simulink model "single_tank"  (R2023b)
settings: Solver=ode45  StartTime=0.0  StopTime=199.9  RelTol=1e-3  EnableMultiTasking=on
values from neighbouring files (symbols this model uses):
  A1 = 0.0154    [INIT.m]
  Cvo = 1.59640*1e-4    (= 0.00015964)    [INIT.m]
  h1c = 0.5    [INIT.m]
  h1c_0 = 0    [INIT.m]
  h1max = 0.6    [INIT.m]
  Ki = 5*1e-6    (= 5e-06)    [INIT.m]
  Kp = 1e-3    (= 0.001)    [INIT.m]
  Qf1 = 1e-4    (= 0.0001)    [INIT.m]    (also in extract_data.m = 5e-5*randn + 1e-4)
  Qf2 = 1e-4    (= 0.0001)    [INIT.m]    (also in extract_data.m = 5e-5*randn + 1e-4)
  Qpmax = 1e-2    (= 0.01)    [INIT.m]
  rate_noise_mQp = 1e-6    (= 1e-06)    [INIT.m]
  rate_noise_mUp = 1e-6    (= 1e-06)    [INIT.m]
  rate_noise_my1 = 1e-6    (= 1e-06)    [INIT.m]
  Te = 1    [INIT.m]
  yo = 0    [INIT.m]
settings Model: Creator=upcnet  LastModifiedBy=Plambeck
settings SolverCC: AlgebraicLoopSolver=TrustRegion
settings DataIOCC: LimitDataPoints=on  SaveFormat=Array  SignalLoggingSaveFormat=ModelDataLogs  ReturnWorkspaceOutputs=off  SignalLoggingName=sigsOut
settings OptimizationCC: BlockReduction=off  BooleanDataType=off  LifeSpan=inf
settings DebuggingCC: SaveWithParameterizedLinksMsg=none  UnderspecifiedInitializationDetection=Classic  MergeDetectMultiDrivingBlocksExec=none  SignalResolutionControl=TryResolveAllWithWarning  MultiTaskDSMMsg=warning  MultiTaskCondExecSysMsg=none  UnconnectedInputMsg=warning  UnconnectedOutputMsg=warning  UnconnectedLineMsg=warning  AllowSymbolicDim=off  SFUnexpectedBacktrackingDiag=warning  SFNoUnconditionalDefaultTransitionDiag=warning  SFExecutionAtInitializationDiag=none  ArithmeticOperatorsInVariantConditions=warning
settings HardwareCC: ProdBitPerPointer=32  ProdBitPerSizeT=32  ProdBitPerPtrDiffT=32  ProdLargestAtomicFloat=None  ProdIntDivRoundTo=Undefined  ProdEndianess=Unspecified  ProdWordSize=32  ProdHWDeviceType=32-bit Generic  TargetUnknown=on
settings ModelReferenceCC: EnableRefExpFcnMdlSchedulingChecks=on  PropagateSignalLabelsOutOfModel=off
settings SFSimCC: SimUseLocalCustomCode=off  CustomCodeUndefinedFunction=UseInterfaceOnly
settings RTWCC: RTWUseLocalCustomCode=off
settings CodeAppCC: StateflowObjectComments=on
settings GRTTargetCC: TargetLangStandard=C89/C90 (ANSI)  CombineOutputUpdateFcns=off  GRTInterface=on
settings ConfigComp: CovMetricSettings=dw  CovSaveCumulativeToWorkspaceVar=on  CovSaveSingleToWorkspaceVar=on  CovExternalEMLEnable=off

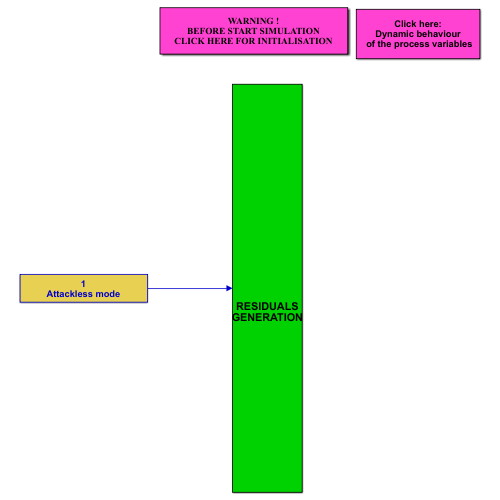
[thumbnail: Simulink's stored preview of the top-level diagram]
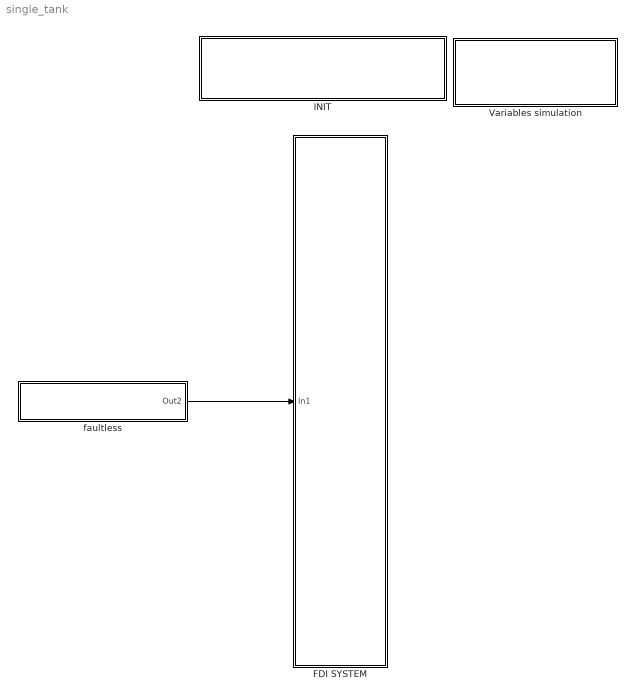
== system single_tank ==
  FDI SYSTEM : Subsystem
      mask Display: disp('\n\n\n\nRESIDUALS\nGENERATION')
  INIT : Subsystem
      settings: OpenFcn=INIT
      mask Display: disp('WARNING !\nBEFORE START SIMULATION\nCLICK HERE FOR INITIALISATION')
  Variables simulation : Subsystem
      mask Display: disp('Click here:\nDynamic behaviour\n of the process variables')
  faultless : Subsystem
      mask Display: disp('1\nAttackless mode')
  wires:
  faultless/1(Out2) -> FDI SYSTEM/1(In1)

== system single_tank/FDI SYSTEM ==
  note: Known
      | variables
  In1 : Inport
  To Workspace1 : ToWorkspace  VariableName=Monit  SampleTime=0.1
  tag scope: outputs=global
  wires:
  In1/1 -> To Workspace1/1, [outputs]

== system single_tank/INIT ==

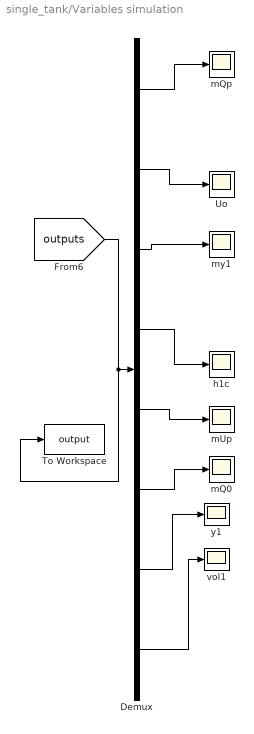
== system single_tank/Variables simulation ==
  Demux : Demux  Outputs=8
      settings: DisplayOption=none
  To Workspace : ToWorkspace  VariableName=output  SampleTime=0.1
  Uo : Scope
  h1c : Scope
  mQ0 : Scope
  mQp : Scope
  mUp : Scope
  my1 : Scope
  vol1 : Scope
  y1 : Scope
  wires:
  [outputs] -> To Workspace/1, Demux/1
  Demux/1 -> mQp/1
  Demux/2 -> Uo/1
  Demux/3 -> my1/1
  Demux/4 -> h1c/1
  Demux/5 -> mUp/1
  Demux/6 -> mQ0/1
  Demux/7 -> y1/1
  Demux/8 -> vol1/1

== system single_tank/faultless ==
  note: mQp
  note: Uo
  note: my1
  note: h1c
  note: mUp
  note: y1
  note: dy
  note: mQ0
  FAULTLESS FAULT : Subsystem
      mask Display: disp('P\nR\nO\nC\nE\nS\nS')
  Mux1 : Mux  Inputs=9
  Out2 : Outport
  wires:
  FAULTLESS FAULT/1(mQp) -> Mux1/1
  FAULTLESS FAULT/2("Uo ") -> Mux1/2
  FAULTLESS FAULT/3(my1) -> Mux1/3
  FAULTLESS FAULT/4(h1c) -> Mux1/4
  FAULTLESS FAULT/5(mUp) -> Mux1/5
  Mux1/1 -> Out2/1
  FAULTLESS FAULT/6(mq0) -> Mux1/6
  FAULTLESS FAULT/7(y1) -> Mux1/7
  FAULTLESS FAULT/8(vol1) -> Mux1/8
  FAULTLESS FAULT/9(dy) -> Mux1/9

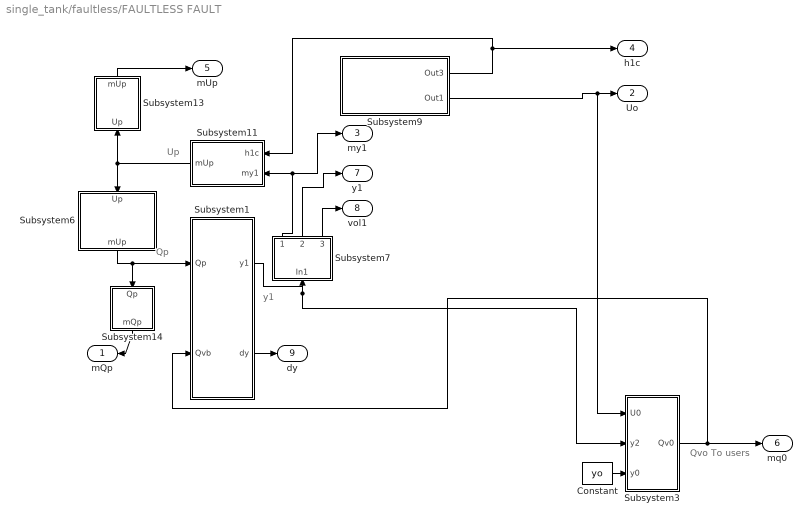
== system single_tank/faultless/FAULTLESS FAULT ==
  note: y1
  note: Up
  note: Qvo
      | To users
  note: Qp
  Constant : Constant  Value=yo
  Subsystem1 : Subsystem
      mask Display: disp('TANK 1')
  Subsystem11 : Subsystem
      mask Display: disp('Controller 1')
  Subsystem13 : Subsystem
      mask Display: disp('Sensor\n Up')
  Subsystem14 : Subsystem
      mask Display: disp('Sensor\n Qp')
  Subsystem3 : Subsystem
      mask Display: disp('Valve O')
  Subsystem6 : Subsystem
      mask Display: disp('Pump')
  Subsystem7 : Subsystem
      mask Display: disp('Sensor\n y1')
  Subsystem9 : Subsystem
      mask Display: disp('OPERATOR\nSET')
  mQp : Outport
  "Uo " : Outport  Port=2
  my1 : Outport  Port=3
  h1c : Outport  Port=4
  mUp : Outport  Port=5
  mq0 : Outport  Port=6
  y1 : Outport  Port=7
  vol1 : Outport  Port=8
  dy : Outport  Port=9
  wires:
  Subsystem1/1(y1) -> Subsystem3/2(y2), Subsystem7/1(In1)
  Subsystem3/1(Qv0) -> Subsystem1/2(Qvb), mq0/1
  Constant/1 -> Subsystem3/3(y0)
  Subsystem13/1(mUp) -> mUp/1
  Subsystem11/1(mUp) -> Subsystem13/1(Up), Subsystem6/1(Up)
  Subsystem9/1(Out3) -> Subsystem11/1(h1c), h1c/1
  Subsystem9/2(Out1) -> "Uo "/1, Subsystem3/1(U0)
  Subsystem7/1(Out5) -> Subsystem11/2(my1), my1/1
  Subsystem14/1(mQp) -> mQp/1
  Subsystem6/1(mUp) -> Subsystem1/1(Qp), Subsystem14/1(Qp)
  Subsystem7/3(Out2) -> vol1/1
  Subsystem7/2(Out1) -> y1/1
  Subsystem1/2(dy) -> dy/1

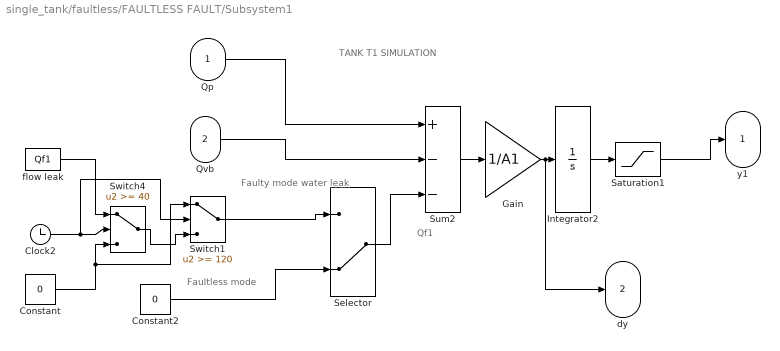
== system single_tank/faultless/FAULTLESS FAULT/Subsystem1 ==
  note: TANK T1 SIMULATION
  note: Qf1
  note: Faultless mode
  note: Faulty mode
      | water leak
  Qp : Inport
  Qvb : Inport  Port=2
  Clock2 : Clock
  Constant : Constant  Value=0
  Constant2 : Constant  Value=0
  Gain : Gain  Gain=1/A1  SaturateOnIntegerOverflow=on  OutDataTypeStr=Inherit: Same as input  ParamDataTypeStr=Inherit: Same as input
  Integrator2 : Integrator  InitialCondition=h1c_0
  Saturation1 : Saturate  UpperLimit=h1max  LowerLimit=0  LinearizeAsGain=off
  Selector : ManualSwitch  CurrentSetting=0
  Sum2 : Sum  Inputs=+--  InputSameDT=on  SaturateOnIntegerOverflow=on  OutDataTypeStr=Inherit: Same as first input
  Switch1 : Switch  Threshold=120
  Switch4 : Switch  Threshold=40
  flow leak : Constant  Value=Qf1
  y1 : Outport  InitialOutput=0
  dy : Outport  Port=2  InitialOutput=0
  wires:
  Sum2/1 -> Gain/1
  Qp/1 -> Sum2/1
  Qvb/1 -> Sum2/2
  Clock2/1 -> Switch4/2, Switch1/2
  flow leak/1 -> Switch4/1
  Constant/1 -> Switch4/3, Switch1/1
  Switch4/1 -> Switch1/3
  Selector/1 -> Sum2/3
  Switch1/1 -> Selector/1
  Constant2/1 -> Selector/2
  Integrator2/1 -> Saturation1/1
  Saturation1/1 -> y1/1
  Gain/1 -> dy/1, Integrator2/1

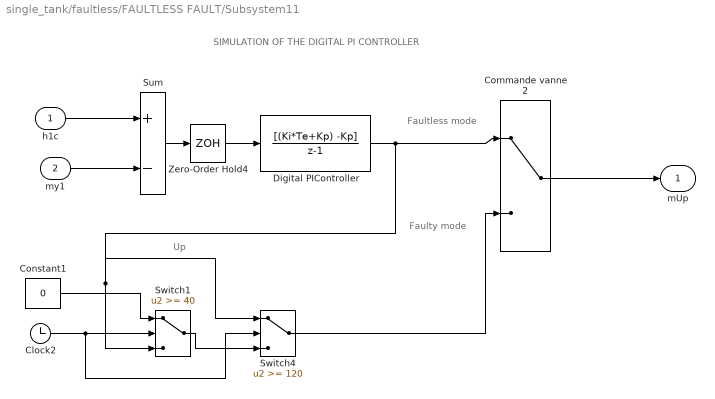
== system single_tank/faultless/FAULTLESS FAULT/Subsystem11 ==
  note: Faultless mode
  note: Faulty mode
  note: Up
  note: SIMULATION OF THE DIGITAL PI CONTROLLER
  h1c : Inport
  my1 : Inport  Port=2
  Clock2 : Clock
  Commande vanne 2 : ManualSwitch
  Constant1 : Constant  Value=0
  Digital PIController : DiscreteTransferFcn  Numerator=[(Ki*Te+Kp) -Kp]  Denominator=[1 -1]  SampleTime=Te
  Sum : Sum  Inputs=+-  InputSameDT=on  SaturateOnIntegerOverflow=on  OutDataTypeStr=Inherit: Same as first input
  Switch1 : Switch  Threshold=40
  Switch4 : Switch  Threshold=120
  Zero-Order Hold4 : ZeroOrderHold  SampleTime=Te
  mUp : Outport  InitialOutput=0
  wires:
  Switch4/1 -> Commande vanne 2/2
  Commande vanne 2/1 -> mUp/1
  Digital PIController/1 -> Switch4/1, Switch1/3, Commande vanne 2/1
  Switch1/1 -> Switch4/3
  Constant1/1 -> Switch1/1
  Clock2/1 -> Switch4/2, Switch1/2
  h1c/1 -> Sum/1
  my1/1 -> Sum/2
  Zero-Order Hold4/1 -> Digital PIController/1
  Sum/1 -> Zero-Order Hold4/1

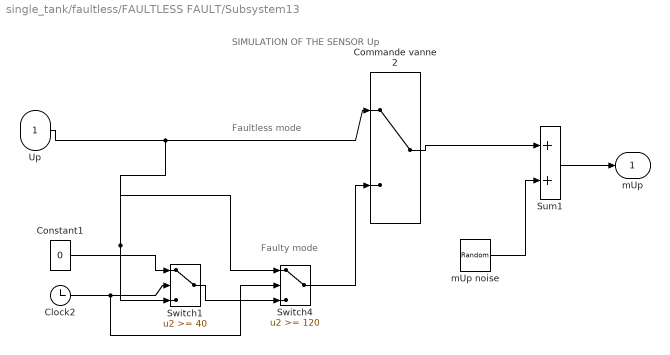
== system single_tank/faultless/FAULTLESS FAULT/Subsystem13 ==
  note: SIMULATION OF THE SENSOR Up
  note: Faultless mode
  note: Faulty mode
  Up : Inport
  Clock2 : Clock
  Commande vanne 2 : ManualSwitch
  Constant1 : Constant  Value=0
  Sum1 : Sum  InputSameDT=on  SaturateOnIntegerOverflow=on  OutDataTypeStr=Inherit: Same as first input
  Switch1 : Switch  Threshold=40
  Switch4 : Switch  Threshold=120
  mUp noise : UniformRandomNumber  Minimum=-rate_noise_mUp  Maximum=rate_noise_mUp  SampleTime=0
  mUp : Outport  InitialOutput=0
  wires:
  Up/1 -> Commande vanne 2/1, Switch1/3, Switch4/1
  Clock2/1 -> Switch1/2, Switch4/2
  Constant1/1 -> Switch1/1
  Switch1/1 -> Switch4/3
  Switch4/1 -> Commande vanne 2/2
  Sum1/1 -> mUp/1
  mUp noise/1 -> Sum1/2
  Commande vanne 2/1 -> Sum1/1

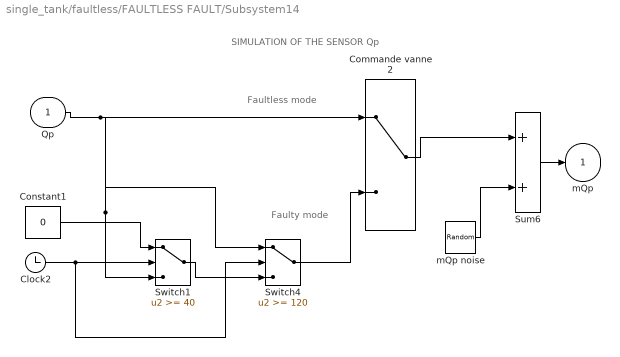
== system single_tank/faultless/FAULTLESS FAULT/Subsystem14 ==
  note: SIMULATION OF THE SENSOR Qp
  note: Faultless mode
  note: Faulty mode
  Qp : Inport
  Clock2 : Clock
  Commande vanne 2 : ManualSwitch
  Constant1 : Constant  Value=0
  Sum6 : Sum  InputSameDT=on  SaturateOnIntegerOverflow=on  OutDataTypeStr=Inherit: Same as first input
  Switch1 : Switch  Threshold=40
  Switch4 : Switch  Threshold=120
  mQp noise : UniformRandomNumber  Minimum=-rate_noise_mQp  Maximum=rate_noise_mQp  SampleTime=0
  mQp : Outport  InitialOutput=0
  wires:
  Sum6/1 -> mQp/1
  Clock2/1 -> Switch1/2, Switch4/2
  Constant1/1 -> Switch1/1
  Switch1/1 -> Switch4/3
  Qp/1 -> Commande vanne 2/1, Switch1/3, Switch4/1
  Commande vanne 2/1 -> Sum6/1
  Switch4/1 -> Commande vanne 2/2
  mQp noise/1 -> Sum6/2

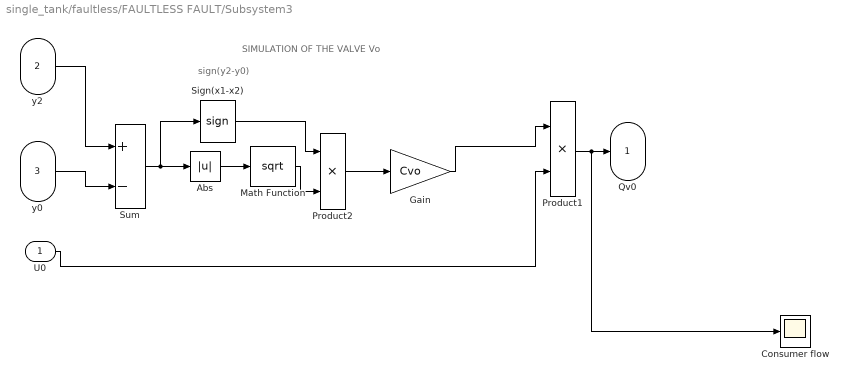
== system single_tank/faultless/FAULTLESS FAULT/Subsystem3 ==
  note: SIMULATION OF THE VALVE Vo
  note: sign(y2-y0)
  U0 : Inport
  y2 : Inport  Port=2
  y0 : Inport  Port=3
  Abs : Abs
  Consumer flow : Scope
  Gain : Gain  Gain=Cvo  SaturateOnIntegerOverflow=on  OutDataTypeStr=Inherit: Same as input  ParamDataTypeStr=Inherit: Same as input
  Math Function : Math  Operator=sqrt  SignedPower=on
  Product1 : Product  InputSameDT=on  SaturateOnIntegerOverflow=on  OutDataTypeStr=Inherit: Same as first input
  Product2 : Product  InputSameDT=on  SaturateOnIntegerOverflow=on  OutDataTypeStr=Inherit: Same as first input
  Sign(x1-x2) : Signum
  Sum : Sum  Inputs=+-  InputSameDT=on  SaturateOnIntegerOverflow=on  OutDataTypeStr=Inherit: Same as first input
  Qv0 : Outport  InitialOutput=0
  wires:
  Product1/1 -> Consumer flow/1, Qv0/1
  Product2/1 -> Gain/1
  y0/1 -> Sum/2
  y2/1 -> Sum/1
  Sign(x1-x2)/1 -> Product2/1
  Math Function/1 -> Product2/2
  Abs/1 -> Math Function/1
  Sum/1 -> Abs/1, Sign(x1-x2)/1
  Gain/1 -> Product1/1
  U0/1 -> Product1/2

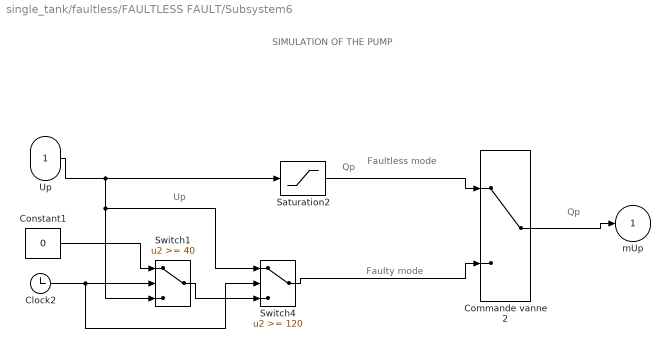
== system single_tank/faultless/FAULTLESS FAULT/Subsystem6 ==
  note: SIMULATION OF THE PUMP
  note: Up
  note: Qp
  note: Qp
  note: Faultless mode
  note: Faulty mode
  Up : Inport
  Clock2 : Clock
  Commande vanne 2 : ManualSwitch
  Constant1 : Constant  Value=0
  Saturation2 : Saturate  UpperLimit=Qpmax  LowerLimit=0  LinearizeAsGain=off
  Switch1 : Switch  Threshold=40
  Switch4 : Switch  Threshold=120
  mUp : Outport  InitialOutput=0
  wires:
  Clock2/1 -> Switch1/2, Switch4/2
  Up/1 -> Switch1/3, Switch4/1, Saturation2/1
  Constant1/1 -> Switch1/1
  Switch1/1 -> Switch4/3
  Commande vanne 2/1 -> mUp/1
  Saturation2/1 -> Commande vanne 2/1
  Switch4/1 -> Commande vanne 2/2

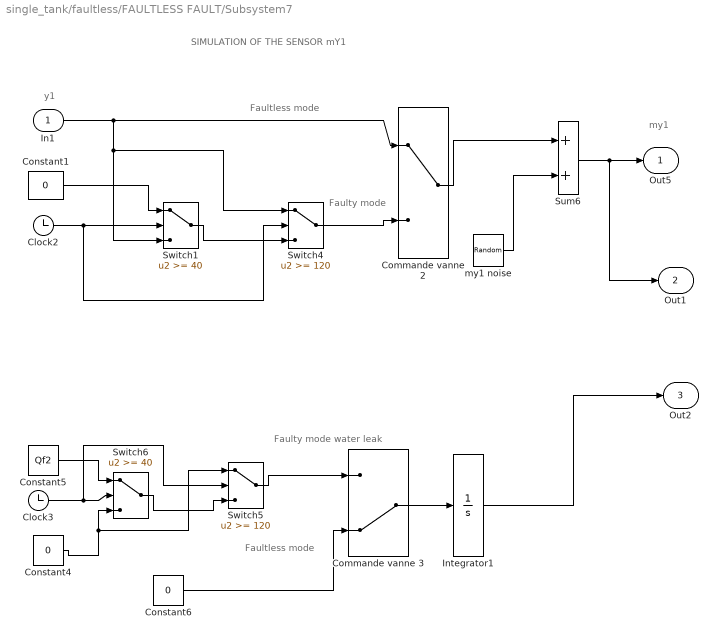
== system single_tank/faultless/FAULTLESS FAULT/Subsystem7 ==
  note: SIMULATION OF THE SENSOR mY1
  note: y1
  note: my1
  note: Faultless mode
  note: Faulty mode
  note: Faultless mode
  note: Faulty mode
      | water leak
  In1 : Inport
  Clock2 : Clock
  Clock3 : Clock
  Commande vanne 2 : ManualSwitch
  Commande vanne 3 : ManualSwitch  CurrentSetting=0
  Constant1 : Constant  Value=0
  Constant4 : Constant  Value=0
  Constant5 : Constant  Value=Qf2
  Constant6 : Constant  Value=0
  Integrator1 : Integrator
  Sum6 : Sum  InputSameDT=on  SaturateOnIntegerOverflow=on  OutDataTypeStr=Inherit: Same as first input
  Switch1 : Switch  Threshold=40
  Switch4 : Switch  Threshold=120
  Switch5 : Switch  Threshold=120
  Switch6 : Switch  Threshold=40
  my1 noise : UniformRandomNumber  Minimum=-rate_noise_my1  Maximum=rate_noise_my1  SampleTime=0
  Out5 : Outport  InitialOutput=0
  Out1 : Outport  Port=2  InitialOutput=0
  Out2 : Outport  Port=3  InitialOutput=0
  wires:
  Clock2/1 -> Switch1/2, Switch4/2
  Constant1/1 -> Switch1/1
  Switch1/1 -> Switch4/3
  Switch4/1 -> Commande vanne 2/2
  In1/1 -> Switch1/3, Switch4/1, Commande vanne 2/1
  Commande vanne 2/1 -> Sum6/1
  my1 noise/1 -> Sum6/2
  Sum6/1 -> Out1/1, Out5/1
  Clock3/1 -> Switch6/2, Switch5/2
  Constant5/1 -> Switch6/1
  Constant4/1 -> Switch6/3, Switch5/1
  Switch6/1 -> Switch5/3
  Switch5/1 -> Commande vanne 3/1
  Constant6/1 -> Commande vanne 3/2
  Integrator1/1 -> Out2/1
  Commande vanne 3/1 -> Integrator1/1

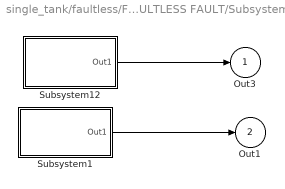
== system single_tank/faultless/FAULTLESS FAULT/Subsystem9 ==
  Subsystem1 : Subsystem
      mask Display: disp('Set \nvalve  V2')
  Subsystem12 : Subsystem
      mask Display: disp('Set\n point h1c')
  Out3 : Outport  InitialOutput=0
  Out1 : Outport  Port=2  InitialOutput=0
  wires:
  Subsystem1/1(Out1) -> Out1/1
  Subsystem12/1(Out1) -> Out3/1

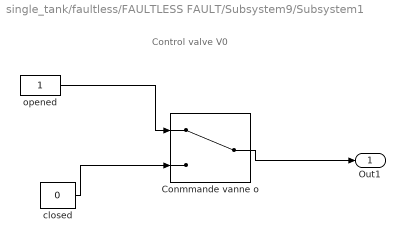
== system single_tank/faultless/FAULTLESS FAULT/Subsystem9/Subsystem1 ==
  note: Control valve V0
  Conmmande vanne o : ManualSwitch
  closed : Constant  Value=0
  opened : Constant
  Out1 : Outport  InitialOutput=0
  wires:
  closed/1 -> Conmmande vanne o/2
  opened/1 -> Conmmande vanne o/1
  Conmmande vanne o/1 -> Out1/1

== system single_tank/faultless/FAULTLESS FAULT/Subsystem9/Subsystem12 ==
  "Set of level of tank 1 " : Step  Time=0  Before=h1c_0  After=h1c  SampleTime=0
  Out1 : Outport
  wires:
  "Set of level of tank 1 "/1 -> Out1/1
